simulink model "parallel_prediction_and_cost_function_6phase"  (R2022a)
settings: Solver=FixedStepDiscrete  StartTime=0.0  StopTime=10.0  RelTol=1e-3
undefined symbols (not defined in the file): f_c, L_d, L_q, L_x, L_y, p, psi_pm, R_ph
libraries: hdlsllib x5
(part 2 of 3)

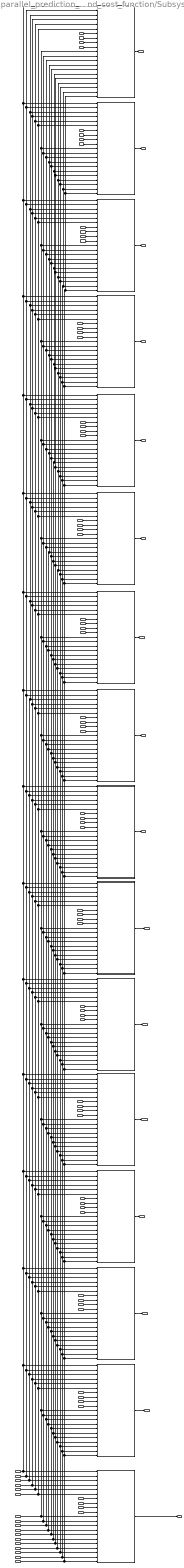
== system parallel_prediction_and_cost_function_6phase/Prediction_and_cost_function/Subsystem ==
  d_phase_voltage_per_switching_state : Inport
  q_phase_voltage_per_switching_state : Inport  Port=2
  x_phase_voltage_per_switching_state : Inport  Port=3
  y_phase_voltage_per_switching_state : Inport  Port=4
  d_phase_voltage_per_switching_state1 : Inport  Port=5
  q_phase_voltage_per_switching_state1 : Inport  Port=6
  x_phase_voltage_per_switching_state1 : Inport  Port=7
  y_phase_voltage_per_switching_state1 : Inport  Port=8
  d_phase_voltage_per_switching_state2 : Inport  Port=9
  q_phase_voltage_per_switching_state2 : Inport  Port=10
  x_phase_voltage_per_switching_state2 : Inport  Port=11
  y_phase_voltage_per_switching_state2 : Inport  Port=12
  d_phase_voltage_per_switching_state3 : Inport  Port=13
  q_phase_voltage_per_switching_state3 : Inport  Port=14
  x_phase_voltage_per_switching_state3 : Inport  Port=15
  y_phase_voltage_per_switching_state3 : Inport  Port=16
  d_phase_voltage_per_switching_state4 : Inport  Port=17
  q_phase_voltage_per_switching_state4 : Inport  Port=18
  x_phase_voltage_per_switching_state4 : Inport  Port=19
  y_phase_voltage_per_switching_state4 : Inport  Port=20
  d_phase_voltage_per_switching_state5 : Inport  Port=21
  q_phase_voltage_per_switching_state5 : Inport  Port=22
  x_phase_voltage_per_switching_state5 : Inport  Port=23
  y_phase_voltage_per_switching_state5 : Inport  Port=24
  d_phase_voltage_per_switching_state6 : Inport  Port=25
  q_phase_voltage_per_switching_state6 : Inport  Port=26
  x_phase_voltage_per_switching_state6 : Inport  Port=27
  y_phase_voltage_per_switching_state6 : Inport  Port=28
  d_phase_voltage_per_switching_state7 : Inport  Port=29
  q_phase_voltage_per_switching_state7 : Inport  Port=30
  x_phase_voltage_per_switching_state7 : Inport  Port=31
  y_phase_voltage_per_switching_state7 : Inport  Port=32
  d_phase_voltage_per_switching_state8 : Inport  Port=33
  q_phase_voltage_per_switching_state8 : Inport  Port=34
  x_phase_voltage_per_switching_state8 : Inport  Port=35
  y_phase_voltage_per_switching_state8 : Inport  Port=36
  d_phase_voltage_per_switching_state9 : Inport  Port=37
  q_phase_voltage_per_switching_state9 : Inport  Port=38
  x_phase_voltage_per_switching_state9 : Inport  Port=39
  y_phase_voltage_per_switching_state9 : Inport  Port=40
  d_phase_voltage_per_switching_state10 : Inport  Port=41
  q_phase_voltage_per_switching_state10 : Inport  Port=42
  x_phase_voltage_per_switching_state10 : Inport  Port=43
  y_phase_voltage_per_switching_state10 : Inport  Port=44
  d_phase_voltage_per_switching_state11 : Inport  Port=45
  q_phase_voltage_per_switching_state11 : Inport  Port=46
  x_phase_voltage_per_switching_state11 : Inport  Port=47
  y_phase_voltage_per_switching_state11 : Inport  Port=48
  d_phase_voltage_per_switching_state12 : Inport  Port=49
  q_phase_voltage_per_switching_state12 : Inport  Port=50
  x_phase_voltage_per_switching_state12 : Inport  Port=51
  y_phase_voltage_per_switching_state12 : Inport  Port=52
  d_phase_voltage_per_switching_state13 : Inport  Port=53
  q_phase_voltage_per_switching_state13 : Inport  Port=54
  x_phase_voltage_per_switching_state13 : Inport  Port=55
  y_phase_voltage_per_switching_state13 : Inport  Port=56
  d_phase_voltage_per_switching_state14 : Inport  Port=57
  q_phase_voltage_per_switching_state14 : Inport  Port=58
  x_phase_voltage_per_switching_state14 : Inport  Port=59
  y_phase_voltage_per_switching_state14 : Inport  Port=60
  SampleTime_div_Ld15 : Inport  Port=61
  SampleTime_div_Lq15 : Inport  Port=62
  SampleTime_div_Lx15 : Inport  Port=63
  SampleTime_div_Ly15 : Inport  Port=64
  id_k_16 : Inport  Port=65
  iq_k_16 : Inport  Port=66
  ix_k_16 : Inport  Port=67
  iy_k_16 : Inport  Port=68
  Rs15 : Inport  Port=69
  omega_el15 : Inport  Port=70
  Lq15 : Inport  Port=71
  Ld15 : Inport  Port=72
  psiPM15 : Inport  Port=73
  d_phase_voltage_per_switching_state15 : Inport  Port=74
  q_phase_voltage_per_switching_state15 : Inport  Port=75
  x_phase_voltage_per_switching_state15 : Inport  Port=76
  y_phase_voltage_per_switching_state15 : Inport  Port=77
  id_ref15 : Inport  Port=78
  iq_ref15 : Inport  Port=79
  ix_ref15 : Inport  Port=80
  iy_ref15 : Inport  Port=81
  Subsystem : Subsystem
  Subsystem1 : Subsystem
  Subsystem10 : Subsystem
  Subsystem11 : Subsystem
  Subsystem12 : Subsystem
  Subsystem13 : Subsystem
  Subsystem14 : Subsystem
  Subsystem15 : Subsystem
  Subsystem2 : Subsystem
  Subsystem3 : Subsystem
  Subsystem4 : Subsystem
  Subsystem5 : Subsystem
  Subsystem6 : Subsystem
  Subsystem7 : Subsystem
  Subsystem8 : Subsystem
  Subsystem9 : Subsystem
  J : Outport
  J1 : Outport  Port=2
  J2 : Outport  Port=3
  J3 : Outport  Port=4
  J4 : Outport  Port=5
  J5 : Outport  Port=6
  J6 : Outport  Port=7
  J7 : Outport  Port=8
  J8 : Outport  Port=9
  J9 : Outport  Port=10
  J10 : Outport  Port=11
  J11 : Outport  Port=12
  J12 : Outport  Port=13
  J13 : Outport  Port=14
  J14 : Outport  Port=15
  J15 : Outport  Port=16
  wires:
  d_phase_voltage_per_switching_state13/1 -> Subsystem2/7(d_phase_voltage_per_switching_state)
  q_phase_voltage_per_switching_state1/1 -> Subsystem14/8(q_phase_voltage_per_switching_state)
  x_phase_voltage_per_switching_state12/1 -> Subsystem3/9(x_phase_voltage_per_switching_state)
  y_phase_voltage_per_switching_state/1 -> Subsystem15/10(y_phase_voltage_per_switching_state)
  y_phase_voltage_per_switching_state2/1 -> Subsystem13/10(y_phase_voltage_per_switching_state)
  d_phase_voltage_per_switching_state1/1 -> Subsystem14/7(d_phase_voltage_per_switching_state)
  x_phase_voltage_per_switching_state1/1 -> Subsystem14/9(x_phase_voltage_per_switching_state)
  y_phase_voltage_per_switching_state7/1 -> Subsystem8/10(y_phase_voltage_per_switching_state)
  d_phase_voltage_per_switching_state3/1 -> Subsystem12/7(d_phase_voltage_per_switching_state)
  d_phase_voltage_per_switching_state6/1 -> Subsystem9/7(d_phase_voltage_per_switching_state)
  x_phase_voltage_per_switching_state9/1 -> Subsystem6/9(x_phase_voltage_per_switching_state)
  d_phase_voltage_per_switching_state/1 -> Subsystem15/7(d_phase_voltage_per_switching_state)
  x_phase_voltage_per_switching_state3/1 -> Subsystem12/9(x_phase_voltage_per_switching_state)
  d_phase_voltage_per_switching_state2/1 -> Subsystem13/7(d_phase_voltage_per_switching_state)
  x_phase_voltage_per_switching_state8/1 -> Subsystem7/9(x_phase_voltage_per_switching_state)
  y_phase_voltage_per_switching_state9/1 -> Subsystem6/10(y_phase_voltage_per_switching_state)
  x_phase_voltage_per_switching_state4/1 -> Subsystem11/9(x_phase_voltage_per_switching_state)
  y_phase_voltage_per_switching_state1/1 -> Subsystem14/10(y_phase_voltage_per_switching_state)
  q_phase_voltage_per_switching_state2/1 -> Subsystem13/8(q_phase_voltage_per_switching_state)
  x_phase_voltage_per_switching_state2/1 -> Subsystem13/9(x_phase_voltage_per_switching_state)
  y_phase_voltage_per_switching_state11/1 -> Subsystem4/10(y_phase_voltage_per_switching_state)
  y_phase_voltage_per_switching_state4/1 -> Subsystem11/10(y_phase_voltage_per_switching_state)
  x_phase_voltage_per_switching_state/1 -> Subsystem15/9(x_phase_voltage_per_switching_state)
  d_phase_voltage_per_switching_state14/1 -> Subsystem1/7(d_phase_voltage_per_switching_state)
  q_phase_voltage_per_switching_state9/1 -> Subsystem6/8(q_phase_voltage_per_switching_state)
  q_phase_voltage_per_switching_state5/1 -> Subsystem10/8(q_phase_voltage_per_switching_state)
  d_phase_voltage_per_switching_state10/1 -> Subsystem5/7(d_phase_voltage_per_switching_state)
  x_phase_voltage_per_switching_state14/1 -> Subsystem1/9(x_phase_voltage_per_switching_state)
  y_phase_voltage_per_switching_state14/1 -> Subsystem1/10(y_phase_voltage_per_switching_state)
  q_phase_voltage_per_switching_state14/1 -> Subsystem1/8(q_phase_voltage_per_switching_state)
  q_phase_voltage_per_switching_state11/1 -> Subsystem4/8(q_phase_voltage_per_switching_state)
  x_phase_voltage_per_switching_state11/1 -> Subsystem4/9(x_phase_voltage_per_switching_state)
  d_phase_voltage_per_switching_state11/1 -> Subsystem4/7(d_phase_voltage_per_switching_state)
  y_phase_voltage_per_switching_state12/1 -> Subsystem3/10(y_phase_voltage_per_switching_state)
  x_phase_voltage_per_switching_state13/1 -> Subsystem2/9(x_phase_voltage_per_switching_state)
  d_phase_voltage_per_switching_state9/1 -> Subsystem6/7(d_phase_voltage_per_switching_state)
  d_phase_voltage_per_switching_state7/1 -> Subsystem8/7(d_phase_voltage_per_switching_state)
  d_phase_voltage_per_switching_state4/1 -> Subsystem11/7(d_phase_voltage_per_switching_state)
  q_phase_voltage_per_switching_state4/1 -> Subsystem11/8(q_phase_voltage_per_switching_state)
  q_phase_voltage_per_switching_state12/1 -> Subsystem3/8(q_phase_voltage_per_switching_state)
  d_phase_voltage_per_switching_state8/1 -> Subsystem7/7(d_phase_voltage_per_switching_state)
  x_phase_voltage_per_switching_state5/1 -> Subsystem10/9(x_phase_voltage_per_switching_state)
  d_phase_voltage_per_switching_state12/1 -> Subsystem3/7(d_phase_voltage_per_switching_state)
  x_phase_voltage_per_switching_state7/1 -> Subsystem8/9(x_phase_voltage_per_switching_state)
  q_phase_voltage_per_switching_state/1 -> Subsystem15/8(q_phase_voltage_per_switching_state)
  d_phase_voltage_per_switching_state5/1 -> Subsystem10/7(d_phase_voltage_per_switching_state)
  q_phase_voltage_per_switching_state13/1 -> Subsystem2/8(q_phase_voltage_per_switching_state)
  y_phase_voltage_per_switching_state5/1 -> Subsystem10/10(y_phase_voltage_per_switching_state)
  q_phase_voltage_per_switching_state6/1 -> Subsystem9/8(q_phase_voltage_per_switching_state)
  y_phase_voltage_per_switching_state6/1 -> Subsystem9/10(y_phase_voltage_per_switching_state)
  x_phase_voltage_per_switching_state6/1 -> Subsystem9/9(x_phase_voltage_per_switching_state)
  y_phase_voltage_per_switching_state8/1 -> Subsystem7/10(y_phase_voltage_per_switching_state)
  q_phase_voltage_per_switching_state8/1 -> Subsystem7/8(q_phase_voltage_per_switching_state)
  y_phase_voltage_per_switching_state13/1 -> Subsystem2/10(y_phase_voltage_per_switching_state)
  q_phase_voltage_per_switching_state7/1 -> Subsystem8/8(q_phase_voltage_per_switching_state)
  x_phase_voltage_per_switching_state10/1 -> Subsystem5/9(x_phase_voltage_per_switching_state)
  q_phase_voltage_per_switching_state10/1 -> Subsystem5/8(q_phase_voltage_per_switching_state)
  y_phase_voltage_per_switching_state10/1 -> Subsystem5/10(y_phase_voltage_per_switching_state)
  y_phase_voltage_per_switching_state3/1 -> Subsystem12/10(y_phase_voltage_per_switching_state)
  q_phase_voltage_per_switching_state3/1 -> Subsystem12/8(q_phase_voltage_per_switching_state)
  id_ref15/1 -> Subsystem15/1(id_ref), Subsystem14/1(id_ref), Subsystem13/1(id_ref), Subsystem12/1(id_ref), Subsystem11/1(id_ref), Subsystem10/1(id_ref), Subsystem9/1(id_ref), Subsystem8/1(id_ref), Subsystem7/1(id_ref), Subsystem6/1(id_ref), Subsystem5/1(id_ref), Subsystem4/1(id_ref), Subsystem3/1(id_ref), Subsystem2/1(id_ref), Subsystem1/1(id_ref), Subsystem/1(id_ref)  "id_ref"
  iq_ref15/1 -> Subsystem/2(iq_ref), Subsystem15/2(iq_ref), Subsystem14/2(iq_ref), Subsystem13/2(iq_ref), Subsystem12/2(iq_ref), Subsystem11/2(iq_ref), Subsystem10/2(iq_ref), Subsystem9/2(iq_ref), Subsystem8/2(iq_ref), Subsystem7/2(iq_ref), Subsystem6/2(iq_ref), Subsystem5/2(iq_ref), Subsystem4/2(iq_ref), Subsystem3/2(iq_ref), Subsystem2/2(iq_ref), Subsystem1/2(iq_ref)  "iq_ref"
  SampleTime_div_Ld15/1 -> Subsystem/3(SampleTime_div_Ld), Subsystem4/3(SampleTime_div_Ld), Subsystem7/3(SampleTime_div_Ld), Subsystem15/3(SampleTime_div_Ld), Subsystem14/3(SampleTime_div_Ld), Subsystem13/3(SampleTime_div_Ld), Subsystem12/3(SampleTime_div_Ld), Subsystem11/3(SampleTime_div_Ld), Subsystem10/3(SampleTime_div_Ld), Subsystem9/3(SampleTime_div_Ld), Subsystem8/3(SampleTime_div_Ld), Subsystem6/3(SampleTime_div_Ld), Subsystem5/3(SampleTime_div_Ld), Subsystem3/3(SampleTime_div_Ld), Subsystem2/3(SampleTime_div_Ld), Subsystem1/3(SampleTime_div_Ld)  "SampleTime_div_Ld"
  SampleTime_div_Lq15/1 -> Subsystem/4(SampleTime_div_Lq), Subsystem4/4(SampleTime_div_Lq), Subsystem15/4(SampleTime_div_Lq), Subsystem14/4(SampleTime_div_Lq), Subsystem13/4(SampleTime_div_Lq), Subsystem12/4(SampleTime_div_Lq), Subsystem11/4(SampleTime_div_Lq), Subsystem10/4(SampleTime_div_Lq), Subsystem9/4(SampleTime_div_Lq), Subsystem8/4(SampleTime_div_Lq), Subsystem7/4(SampleTime_div_Lq), Subsystem6/4(SampleTime_div_Lq), Subsystem5/4(SampleTime_div_Lq), Subsystem3/4(SampleTime_div_Lq), Subsystem2/4(SampleTime_div_Lq), Subsystem1/4(SampleTime_div_Lq)  "SampleTime_div_Lq"
  SampleTime_div_Lx15/1 -> Subsystem/5(SampleTime_div_Lx), Subsystem15/5(SampleTime_div_Lx), Subsystem14/5(SampleTime_div_Lx), Subsystem13/5(SampleTime_div_Lx), Subsystem12/5(SampleTime_div_Lx), Subsystem11/5(SampleTime_div_Lx), Subsystem10/5(SampleTime_div_Lx), Subsystem9/5(SampleTime_div_Lx), Subsystem8/5(SampleTime_div_Lx), Subsystem7/5(SampleTime_div_Lx), Subsystem6/5(SampleTime_div_Lx), Subsystem5/5(SampleTime_div_Lx), Subsystem4/5(SampleTime_div_Lx), Subsystem3/5(SampleTime_div_Lx), Subsystem2/5(SampleTime_div_Lx), Subsystem1/5(SampleTime_div_Lx)  "SampleTime_div_Lx"
  SampleTime_div_Ly15/1 -> Subsystem/6(SampleTime_div_Ly), Subsystem15/6(SampleTime_div_Ly), Subsystem14/6(SampleTime_div_Ly), Subsystem13/6(SampleTime_div_Ly), Subsystem12/6(SampleTime_div_Ly), Subsystem11/6(SampleTime_div_Ly), Subsystem10/6(SampleTime_div_Ly), Subsystem9/6(SampleTime_div_Ly), Subsystem8/6(SampleTime_div_Ly), Subsystem7/6(SampleTime_div_Ly), Subsystem6/6(SampleTime_div_Ly), Subsystem5/6(SampleTime_div_Ly), Subsystem4/6(SampleTime_div_Ly), Subsystem3/6(SampleTime_div_Ly), Subsystem2/6(SampleTime_div_Ly), Subsystem1/6(SampleTime_div_Ly)  "SampleTime_div_Ly"
  d_phase_voltage_per_switching_state15/1 -> Subsystem/7(d_phase_voltage_per_switching_state)
  q_phase_voltage_per_switching_state15/1 -> Subsystem/8(q_phase_voltage_per_switching_state)
  x_phase_voltage_per_switching_state15/1 -> Subsystem/9(x_phase_voltage_per_switching_state)
  y_phase_voltage_per_switching_state15/1 -> Subsystem/10(y_phase_voltage_per_switching_state)
  ix_ref15/1 -> Subsystem/11(ix_ref), Subsystem15/11(ix_ref), Subsystem14/11(ix_ref), Subsystem13/11(ix_ref), Subsystem12/11(ix_ref), Subsystem11/11(ix_ref), Subsystem10/11(ix_ref), Subsystem9/11(ix_ref), Subsystem8/11(ix_ref), Subsystem7/11(ix_ref), Subsystem6/11(ix_ref), Subsystem5/11(ix_ref), Subsystem4/11(ix_ref), Subsystem3/11(ix_ref), Subsystem2/11(ix_ref), Subsystem1/11(ix_ref)  "ix_ref"
  id_k_16/1 -> Subsystem/12(id_k), Subsystem15/12(id_k), Subsystem14/12(id_k), Subsystem13/12(id_k), Subsystem12/12(id_k), Subsystem11/12(id_k), Subsystem10/12(id_k), Subsystem9/12(id_k), Subsystem8/12(id_k), Subsystem7/12(id_k), Subsystem6/12(id_k), Subsystem5/12(id_k), Subsystem4/12(id_k), Subsystem3/12(id_k), Subsystem2/12(id_k), Subsystem1/12(id_k)  "id_k"
  iq_k_16/1 -> Subsystem/13(iq_k), Subsystem15/13(iq_k), Subsystem14/13(iq_k), Subsystem13/13(iq_k), Subsystem12/13(iq_k), Subsystem11/13(iq_k), Subsystem10/13(iq_k), Subsystem9/13(iq_k), Subsystem8/13(iq_k), Subsystem7/13(iq_k), Subsystem6/13(iq_k), Subsystem5/13(iq_k), Subsystem4/13(iq_k), Subsystem3/13(iq_k), Subsystem2/13(iq_k), Subsystem1/13(iq_k)  "iq_k"
  ix_k_16/1 -> Subsystem/14(ix_k), Subsystem15/14(ix_k), Subsystem14/14(ix_k), Subsystem13/14(ix_k), Subsystem12/14(ix_k), Subsystem11/14(ix_k), Subsystem10/14(ix_k), Subsystem9/14(ix_k), Subsystem8/14(ix_k), Subsystem7/14(ix_k), Subsystem6/14(ix_k), Subsystem5/14(ix_k), Subsystem4/14(ix_k), Subsystem3/14(ix_k), Subsystem2/14(ix_k), Subsystem1/14(ix_k)  "ix_k"
  iy_k_16/1 -> Subsystem/15(iy_k), Subsystem15/15(iy_k), Subsystem14/15(iy_k), Subsystem13/15(iy_k), Subsystem12/15(iy_k), Subsystem11/15(iy_k), Subsystem10/15(iy_k), Subsystem9/15(iy_k), Subsystem8/15(iy_k), Subsystem7/15(iy_k), Subsystem6/15(iy_k), Subsystem5/15(iy_k), Subsystem4/15(iy_k), Subsystem3/15(iy_k), Subsystem2/15(iy_k), Subsystem1/15(iy_k)  "iy_k"
  psiPM15/1 -> Subsystem/16(psiPM), Subsystem10/16(psiPM), Subsystem15/16(psiPM), Subsystem14/16(psiPM), Subsystem13/16(psiPM), Subsystem12/16(psiPM), Subsystem11/16(psiPM), Subsystem9/16(psiPM), Subsystem8/16(psiPM), Subsystem7/16(psiPM), Subsystem6/16(psiPM), Subsystem5/16(psiPM), Subsystem4/16(psiPM), Subsystem3/16(psiPM), Subsystem2/16(psiPM), Subsystem1/16(psiPM)  "psiPM"
  Lq15/1 -> Subsystem/17(Lq), Subsystem15/17(Lq), Subsystem14/17(Lq), Subsystem13/17(Lq), Subsystem12/17(Lq), Subsystem11/17(Lq), Subsystem10/17(Lq), Subsystem9/17(Lq), Subsystem8/17(Lq), Subsystem7/17(Lq), Subsystem6/17(Lq), Subsystem5/17(Lq), Subsystem4/17(Lq), Subsystem3/17(Lq), Subsystem2/17(Lq), Subsystem1/17(Lq)  "Lq"
  iy_ref15/1 -> Subsystem/18(iy_ref), Subsystem1/18(iy_ref), Subsystem6/18(iy_ref), Subsystem15/18(iy_ref), Subsystem14/18(iy_ref), Subsystem13/18(iy_ref), Subsystem12/18(iy_ref), Subsystem11/18(iy_ref), Subsystem10/18(iy_ref), Subsystem9/18(iy_ref), Subsystem8/18(iy_ref), Subsystem7/18(iy_ref), Subsystem5/18(iy_ref), Subsystem4/18(iy_ref), Subsystem3/18(iy_ref), Subsystem2/18(iy_ref)  "iy_ref"
  Ld15/1 -> Subsystem/19(Ld), Subsystem1/19(Ld), Subsystem15/19(Ld), Subsystem14/19(Ld), Subsystem13/19(Ld), Subsystem12/19(Ld), Subsystem11/19(Ld), Subsystem10/19(Ld), Subsystem9/19(Ld), Subsystem8/19(Ld), Subsystem7/19(Ld), Subsystem6/19(Ld), Subsystem5/19(Ld), Subsystem4/19(Ld), Subsystem3/19(Ld), Subsystem2/19(Ld)  "Ld"
  Rs15/1 -> Subsystem/20(Rs), Subsystem7/20(Rs), Subsystem15/20(Rs), Subsystem14/20(Rs), Subsystem13/20(Rs), Subsystem12/20(Rs), Subsystem11/20(Rs), Subsystem10/20(Rs), Subsystem9/20(Rs), Subsystem8/20(Rs), Subsystem6/20(Rs), Subsystem5/20(Rs), Subsystem4/20(Rs), Subsystem3/20(Rs), Subsystem2/20(Rs), Subsystem1/20(Rs)  "Rs"
  omega_el15/1 -> Subsystem/21(omega_el), Subsystem15/21(omega_el), Subsystem14/21(omega_el), Subsystem13/21(omega_el), Subsystem12/21(omega_el), Subsystem11/21(omega_el), Subsystem10/21(omega_el), Subsystem9/21(omega_el), Subsystem8/21(omega_el), Subsystem7/21(omega_el), Subsystem6/21(omega_el), Subsystem5/21(omega_el), Subsystem4/21(omega_el), Subsystem3/21(omega_el), Subsystem2/21(omega_el), Subsystem1/21(omega_el)  "omega_el"
  Subsystem/1(J15) -> J15/1
  Subsystem1/1(J) -> J14/1
  Subsystem2/1(J) -> J13/1
  Subsystem3/1(J) -> J12/1
  Subsystem4/1(J) -> J11/1
  Subsystem5/1(J) -> J10/1
  Subsystem6/1(J) -> J9/1
  Subsystem7/1(J) -> J8/1
  Subsystem8/1(J) -> J7/1
  Subsystem9/1(J) -> J6/1
  Subsystem10/1(J) -> J5/1
  Subsystem11/1(J) -> J4/1
  Subsystem12/1(J) -> J3/1
  Subsystem13/1(J) -> J2/1
  Subsystem14/1(J) -> J1/1
  Subsystem15/1(J) -> J/1

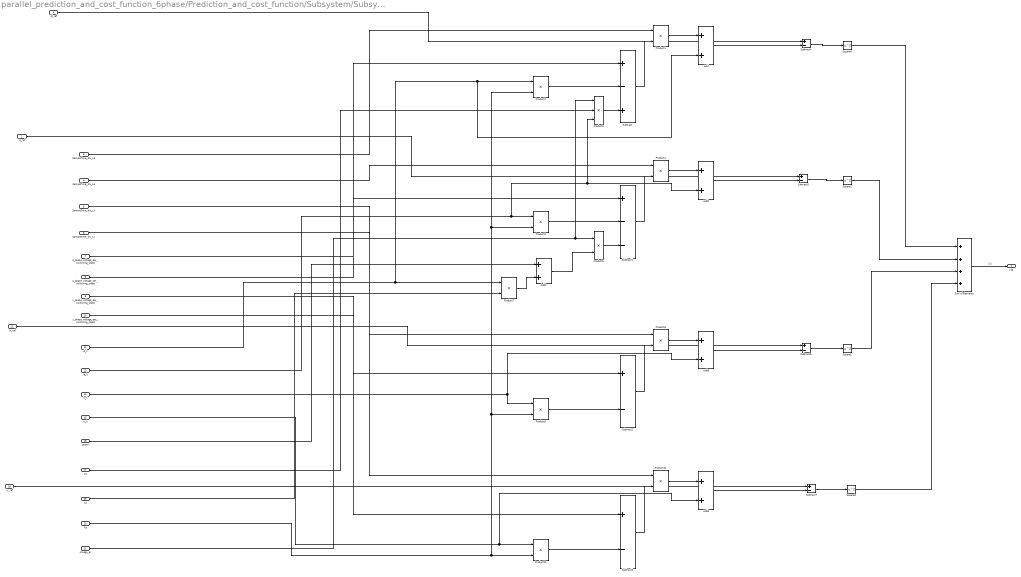
== system parallel_prediction_and_cost_function_6phase/Prediction_and_cost_function/Subsystem/Subsystem ==
  id_ref : Inport
  iq_ref : Inport  Port=2
  SampleTime_div_Ld : Inport  Port=3
  SampleTime_div_Lq : Inport  Port=4
  SampleTime_div_Lx : Inport  Port=5
  SampleTime_div_Ly : Inport  Port=6
  d_phase_voltage_per_switching_state : Inport  Port=7
  q_phase_voltage_per_switching_state : Inport  Port=8
  x_phase_voltage_per_switching_state : Inport  Port=9
  y_phase_voltage_per_switching_state : Inport  Port=10
  ix_ref : Inport  Port=11
  id_k : Inport  Port=12
  iq_k : Inport  Port=13
  ix_k : Inport  Port=14
  iy_k : Inport  Port=15
  psiPM : Inport  Port=16
  Lq : Inport  Port=17
  iy_ref : Inport  Port=18
  Ld : Inport  Port=19
  Rs : Inport  Port=20
  omega_el : Inport  Port=21
  Add{,1,3..4} (4 alike) : Sum  OutDataTypeStr=single
  Add2 : Sum
  Product{1..2,4..11} (10 alike) : Product  OutDataTypeStr=single
  Product3 : Product  Inputs=3  OutDataTypeStr=single
  Square{1..4} (4 alike) : Math  Operator=square  SignedPower=on  RndMeth=Zero
  Subtract : Sum  Inputs=+-+  OutDataTypeStr=single
  Subtract1 : Sum  Inputs=+--  OutDataTypeStr=single
  Subtract2 : Sum  Inputs=+-  OutDataTypeStr=single
  Subtract3 : Sum  Inputs=+-  OutDataTypeStr=single
  Subtract{4..7} (4 alike) : Sum  Inputs=+-
  Sum of Elements : Sum  Inputs=++++
  J15 : Outport
  wires:
  Add1/1 -> Subtract5/2
  q_phase_voltage_per_switching_state/1 -> Subtract1/1
  ix_ref/1 -> Subtract6/1
  omega_el/1 -> Product3/1, Product6/1
  Product5/1 -> Subtract1/2
  iq_k/1 -> Product3/3, Add1/2, Product5/1
  iy_k/1 -> Add4/2, Product11/1
  Add2/1 -> Product6/2
  Lq/1 -> Product3/2
  Add4/1 -> Subtract7/2
  Subtract2/1 -> Product8/2
  SampleTime_div_Ly/1 -> Product10/1
  Rs/1 -> Product9/2, Product2/2, Product5/2, Product11/2
  Product9/1 -> Subtract2/2
  Product8/1 -> Add3/1
  Product7/1 -> Add2/2
  id_k/1 -> Add/2, Product2/1, Product7/1
  x_phase_voltage_per_switching_state/1 -> Subtract2/1
  Add3/1 -> Subtract6/2
  Add/1 -> Subtract4/2
  Product11/1 -> Subtract3/2
  Product6/1 -> Subtract1/3
  Subtract1/1 -> Product4/2
  Product1/1 -> Add/1
  Product10/1 -> Add4/1
  Product4/1 -> Add1/1
  SampleTime_div_Ld/1 -> Product1/1
  y_phase_voltage_per_switching_state/1 -> Subtract3/1
  Product2/1 -> Subtract/2
  Subtract5/1 -> Square1/1
  Product3/1 -> Subtract/3
  SampleTime_div_Lq/1 -> Product4/1
  Subtract/1 -> Product1/2
  Subtract3/1 -> Product10/2
  Sum of Elements/1 -> J15/1  "J15"
  psiPM/1 -> Add2/1
  id_ref/1 -> Subtract4/1
  Subtract6/1 -> Square2/1
  Ld/1 -> Product7/2
  iy_ref/1 -> Subtract7/1
  ix_k/1 -> Add3/2, Product9/1
  Subtract4/1 -> Square4/1
  Subtract7/1 -> Square3/1
  iq_ref/1 -> Subtract5/1
  SampleTime_div_Lx/1 -> Product8/1
  d_phase_voltage_per_switching_state/1 -> Subtract/1
  Square3/1 -> Sum of Elements/4
  Square2/1 -> Sum of Elements/3
  Square1/1 -> Sum of Elements/2
  Square4/1 -> Sum of Elements/1

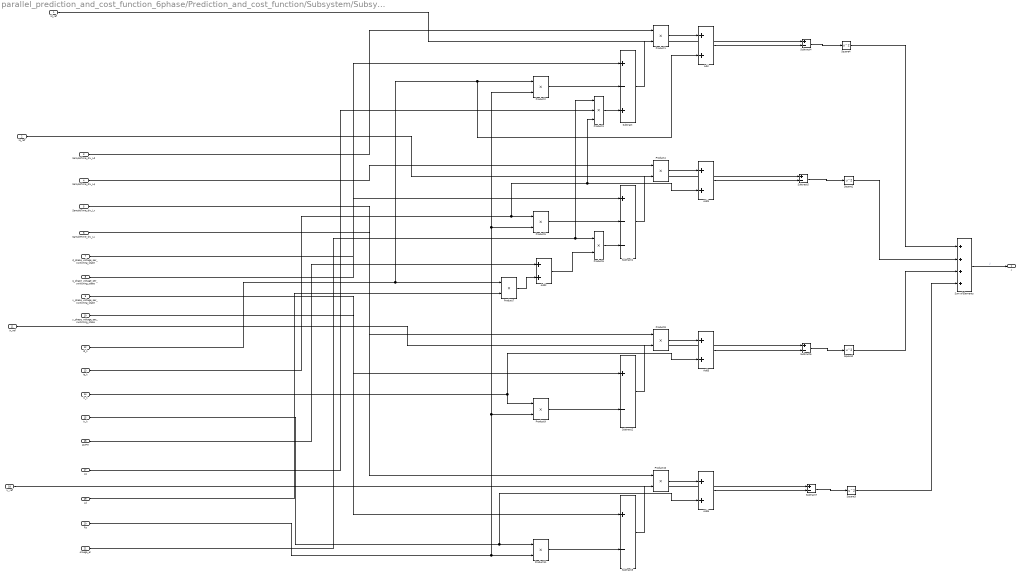
== system parallel_prediction_and_cost_function_6phase/Prediction_and_cost_function/Subsystem/Subsystem1 ==
  id_ref : Inport
  iq_ref : Inport  Port=2
  SampleTime_div_Ld : Inport  Port=3
  SampleTime_div_Lq : Inport  Port=4
  SampleTime_div_Lx : Inport  Port=5
  SampleTime_div_Ly : Inport  Port=6
  d_phase_voltage_per_switching_state : Inport  Port=7
  q_phase_voltage_per_switching_state : Inport  Port=8
  x_phase_voltage_per_switching_state : Inport  Port=9
  y_phase_voltage_per_switching_state : Inport  Port=10
  ix_ref : Inport  Port=11
  id_k : Inport  Port=12
  iq_k : Inport  Port=13
  ix_k : Inport  Port=14
  iy_k : Inport  Port=15
  psiPM : Inport  Port=16
  Lq : Inport  Port=17
  iy_ref : Inport  Port=18
  Ld : Inport  Port=19
  Rs : Inport  Port=20
  omega_el : Inport  Port=21
  Add{,1,3..4} (4 alike) : Sum  OutDataTypeStr=single
  Add2 : Sum
  Product{1..2,4..11} (10 alike) : Product  OutDataTypeStr=single
  Product3 : Product  Inputs=3  OutDataTypeStr=single
  Square{1..4} (4 alike) : Math  Operator=square  SignedPower=on  RndMeth=Zero
  Subtract : Sum  Inputs=+-+  OutDataTypeStr=single
  Subtract1 : Sum  Inputs=+--  OutDataTypeStr=single
  Subtract2 : Sum  Inputs=+-  OutDataTypeStr=single
  Subtract3 : Sum  Inputs=+-  OutDataTypeStr=single
  Subtract{4..7} (4 alike) : Sum  Inputs=+-
  Sum of Elements : Sum  Inputs=++++
  J : Outport
  wires:
  Add1/1 -> Subtract5/2
  q_phase_voltage_per_switching_state/1 -> Subtract1/1
  ix_ref/1 -> Subtract6/1
  omega_el/1 -> Product3/1, Product6/1
  Product5/1 -> Subtract1/2
  iq_k/1 -> Product3/3, Add1/2, Product5/1
  iy_k/1 -> Add4/2, Product11/1
  Add2/1 -> Product6/2
  Lq/1 -> Product3/2
  Add4/1 -> Subtract7/2
  Subtract2/1 -> Product8/2
  SampleTime_div_Ly/1 -> Product10/1
  Rs/1 -> Product9/2, Product2/2, Product5/2, Product11/2
  Product9/1 -> Subtract2/2
  Product8/1 -> Add3/1
  Product7/1 -> Add2/2
  id_k/1 -> Add/2, Product2/1, Product7/1
  x_phase_voltage_per_switching_state/1 -> Subtract2/1
  Add3/1 -> Subtract6/2
  Add/1 -> Subtract4/2
  Product11/1 -> Subtract3/2
  Product6/1 -> Subtract1/3
  Subtract1/1 -> Product4/2
  Product1/1 -> Add/1
  Product10/1 -> Add4/1
  Product4/1 -> Add1/1
  SampleTime_div_Ld/1 -> Product1/1
  y_phase_voltage_per_switching_state/1 -> Subtract3/1
  Product2/1 -> Subtract/2
  Subtract5/1 -> Square1/1
  Product3/1 -> Subtract/3
  SampleTime_div_Lq/1 -> Product4/1
  Subtract/1 -> Product1/2
  Subtract3/1 -> Product10/2
  Sum of Elements/1 -> J/1  "J"
  psiPM/1 -> Add2/1
  id_ref/1 -> Subtract4/1
  Subtract6/1 -> Square2/1
  Ld/1 -> Product7/2
  iy_ref/1 -> Subtract7/1
  ix_k/1 -> Add3/2, Product9/1
  Subtract4/1 -> Square4/1
  Subtract7/1 -> Square3/1
  iq_ref/1 -> Subtract5/1
  SampleTime_div_Lx/1 -> Product8/1
  d_phase_voltage_per_switching_state/1 -> Subtract/1
  Square3/1 -> Sum of Elements/4
  Square2/1 -> Sum of Elements/3
  Square1/1 -> Sum of Elements/2
  Square4/1 -> Sum of Elements/1

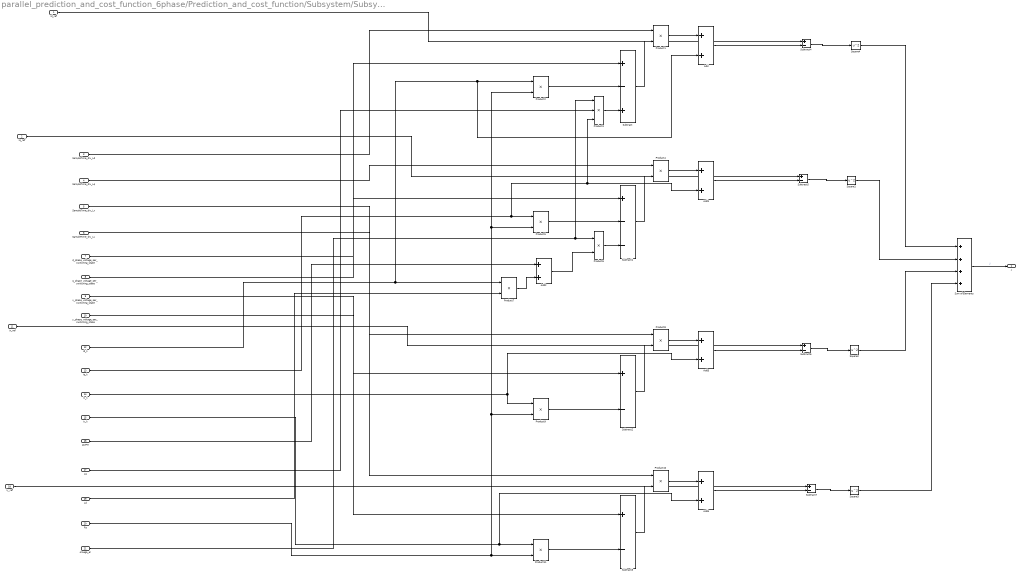
== system parallel_prediction_and_cost_function_6phase/Prediction_and_cost_function/Subsystem/Subsystem10 ==
  id_ref : Inport
  iq_ref : Inport  Port=2
  SampleTime_div_Ld : Inport  Port=3
  SampleTime_div_Lq : Inport  Port=4
  SampleTime_div_Lx : Inport  Port=5
  SampleTime_div_Ly : Inport  Port=6
  d_phase_voltage_per_switching_state : Inport  Port=7
  q_phase_voltage_per_switching_state : Inport  Port=8
  x_phase_voltage_per_switching_state : Inport  Port=9
  y_phase_voltage_per_switching_state : Inport  Port=10
  ix_ref : Inport  Port=11
  id_k : Inport  Port=12
  iq_k : Inport  Port=13
  ix_k : Inport  Port=14
  iy_k : Inport  Port=15
  psiPM : Inport  Port=16
  Lq : Inport  Port=17
  iy_ref : Inport  Port=18
  Ld : Inport  Port=19
  Rs : Inport  Port=20
  omega_el : Inport  Port=21
  Add{,1,3..4} (4 alike) : Sum  OutDataTypeStr=single
  Add2 : Sum
  Product{1..2,4..11} (10 alike) : Product  OutDataTypeStr=single
  Product3 : Product  Inputs=3  OutDataTypeStr=single
  Square{1..4} (4 alike) : Math  Operator=square  SignedPower=on  RndMeth=Zero
  Subtract : Sum  Inputs=+-+  OutDataTypeStr=single
  Subtract1 : Sum  Inputs=+--  OutDataTypeStr=single
  Subtract2 : Sum  Inputs=+-  OutDataTypeStr=single
  Subtract3 : Sum  Inputs=+-  OutDataTypeStr=single
  Subtract{4..7} (4 alike) : Sum  Inputs=+-
  Sum of Elements : Sum  Inputs=++++
  J : Outport
  wires:
  Add1/1 -> Subtract5/2
  q_phase_voltage_per_switching_state/1 -> Subtract1/1
  ix_ref/1 -> Subtract6/1
  omega_el/1 -> Product3/1, Product6/1
  Product5/1 -> Subtract1/2
  iq_k/1 -> Product3/3, Add1/2, Product5/1
  iy_k/1 -> Add4/2, Product11/1
  Add2/1 -> Product6/2
  Lq/1 -> Product3/2
  Add4/1 -> Subtract7/2
  Subtract2/1 -> Product8/2
  SampleTime_div_Ly/1 -> Product10/1
  Rs/1 -> Product9/2, Product2/2, Product5/2, Product11/2
  Product9/1 -> Subtract2/2
  Product8/1 -> Add3/1
  Product7/1 -> Add2/2
  id_k/1 -> Add/2, Product2/1, Product7/1
  x_phase_voltage_per_switching_state/1 -> Subtract2/1
  Add3/1 -> Subtract6/2
  Add/1 -> Subtract4/2
  Product11/1 -> Subtract3/2
  Product6/1 -> Subtract1/3
  Subtract1/1 -> Product4/2
  Product1/1 -> Add/1
  Product10/1 -> Add4/1
  Product4/1 -> Add1/1
  SampleTime_div_Ld/1 -> Product1/1
  y_phase_voltage_per_switching_state/1 -> Subtract3/1
  Product2/1 -> Subtract/2
  Subtract5/1 -> Square1/1
  Product3/1 -> Subtract/3
  SampleTime_div_Lq/1 -> Product4/1
  Subtract/1 -> Product1/2
  Subtract3/1 -> Product10/2
  Sum of Elements/1 -> J/1  "J"
  psiPM/1 -> Add2/1
  id_ref/1 -> Subtract4/1
  Subtract6/1 -> Square2/1
  Ld/1 -> Product7/2
  iy_ref/1 -> Subtract7/1
  ix_k/1 -> Add3/2, Product9/1
  Subtract4/1 -> Square4/1
  Subtract7/1 -> Square3/1
  iq_ref/1 -> Subtract5/1
  SampleTime_div_Lx/1 -> Product8/1
  d_phase_voltage_per_switching_state/1 -> Subtract/1
  Square3/1 -> Sum of Elements/4
  Square2/1 -> Sum of Elements/3
  Square1/1 -> Sum of Elements/2
  Square4/1 -> Sum of Elements/1

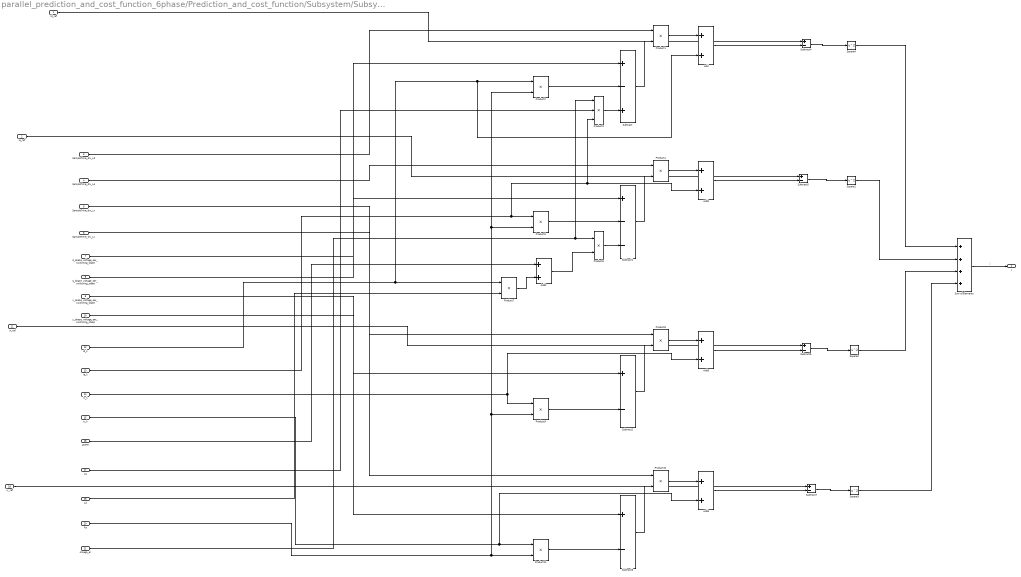
== system parallel_prediction_and_cost_function_6phase/Prediction_and_cost_function/Subsystem/Subsystem11 ==
  id_ref : Inport
  iq_ref : Inport  Port=2
  SampleTime_div_Ld : Inport  Port=3
  SampleTime_div_Lq : Inport  Port=4
  SampleTime_div_Lx : Inport  Port=5
  SampleTime_div_Ly : Inport  Port=6
  d_phase_voltage_per_switching_state : Inport  Port=7
  q_phase_voltage_per_switching_state : Inport  Port=8
  x_phase_voltage_per_switching_state : Inport  Port=9
  y_phase_voltage_per_switching_state : Inport  Port=10
  ix_ref : Inport  Port=11
  id_k : Inport  Port=12
  iq_k : Inport  Port=13
  ix_k : Inport  Port=14
  iy_k : Inport  Port=15
  psiPM : Inport  Port=16
  Lq : Inport  Port=17
  iy_ref : Inport  Port=18
  Ld : Inport  Port=19
  Rs : Inport  Port=20
  omega_el : Inport  Port=21
  Add{,1,3..4} (4 alike) : Sum  OutDataTypeStr=single
  Add2 : Sum
  Product{1..2,4..11} (10 alike) : Product  OutDataTypeStr=single
  Product3 : Product  Inputs=3  OutDataTypeStr=single
  Square{1..4} (4 alike) : Math  Operator=square  SignedPower=on  RndMeth=Zero
  Subtract : Sum  Inputs=+-+  OutDataTypeStr=single
  Subtract1 : Sum  Inputs=+--  OutDataTypeStr=single
  Subtract2 : Sum  Inputs=+-  OutDataTypeStr=single
  Subtract3 : Sum  Inputs=+-  OutDataTypeStr=single
  Subtract{4..7} (4 alike) : Sum  Inputs=+-
  Sum of Elements : Sum  Inputs=++++
  J : Outport
  wires:
  Add1/1 -> Subtract5/2
  q_phase_voltage_per_switching_state/1 -> Subtract1/1
  ix_ref/1 -> Subtract6/1
  omega_el/1 -> Product3/1, Product6/1
  Product5/1 -> Subtract1/2
  iq_k/1 -> Product3/3, Add1/2, Product5/1
  iy_k/1 -> Add4/2, Product11/1
  Add2/1 -> Product6/2
  Lq/1 -> Product3/2
  Add4/1 -> Subtract7/2
  Subtract2/1 -> Product8/2
  SampleTime_div_Ly/1 -> Product10/1
  Rs/1 -> Product9/2, Product2/2, Product5/2, Product11/2
  Product9/1 -> Subtract2/2
  Product8/1 -> Add3/1
  Product7/1 -> Add2/2
  id_k/1 -> Add/2, Product2/1, Product7/1
  x_phase_voltage_per_switching_state/1 -> Subtract2/1
  Add3/1 -> Subtract6/2
  Add/1 -> Subtract4/2
  Product11/1 -> Subtract3/2
  Product6/1 -> Subtract1/3
  Subtract1/1 -> Product4/2
  Product1/1 -> Add/1
  Product10/1 -> Add4/1
  Product4/1 -> Add1/1
  SampleTime_div_Ld/1 -> Product1/1
  y_phase_voltage_per_switching_state/1 -> Subtract3/1
  Product2/1 -> Subtract/2
  Subtract5/1 -> Square1/1
  Product3/1 -> Subtract/3
  SampleTime_div_Lq/1 -> Product4/1
  Subtract/1 -> Product1/2
  Subtract3/1 -> Product10/2
  Sum of Elements/1 -> J/1  "J"
  psiPM/1 -> Add2/1
  id_ref/1 -> Subtract4/1
  Subtract6/1 -> Square2/1
  Ld/1 -> Product7/2
  iy_ref/1 -> Subtract7/1
  ix_k/1 -> Add3/2, Product9/1
  Subtract4/1 -> Square4/1
  Subtract7/1 -> Square3/1
  iq_ref/1 -> Subtract5/1
  SampleTime_div_Lx/1 -> Product8/1
  d_phase_voltage_per_switching_state/1 -> Subtract/1
  Square3/1 -> Sum of Elements/4
  Square2/1 -> Sum of Elements/3
  Square1/1 -> Sum of Elements/2
  Square4/1 -> Sum of Elements/1

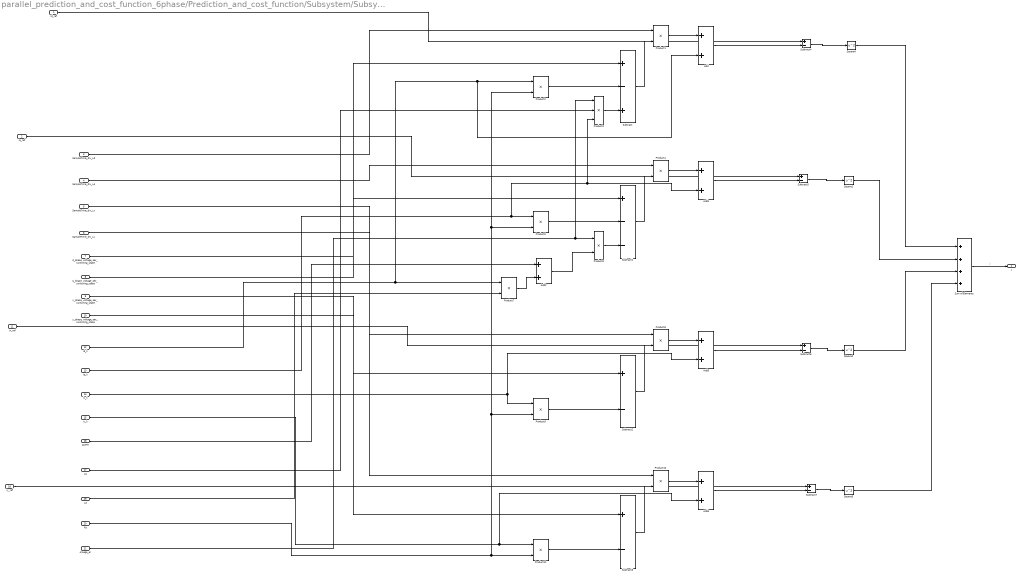
== system parallel_prediction_and_cost_function_6phase/Prediction_and_cost_function/Subsystem/Subsystem12 ==
  id_ref : Inport
  iq_ref : Inport  Port=2
  SampleTime_div_Ld : Inport  Port=3
  SampleTime_div_Lq : Inport  Port=4
  SampleTime_div_Lx : Inport  Port=5
  SampleTime_div_Ly : Inport  Port=6
  d_phase_voltage_per_switching_state : Inport  Port=7
  q_phase_voltage_per_switching_state : Inport  Port=8
  x_phase_voltage_per_switching_state : Inport  Port=9
  y_phase_voltage_per_switching_state : Inport  Port=10
  ix_ref : Inport  Port=11
  id_k : Inport  Port=12
  iq_k : Inport  Port=13
  ix_k : Inport  Port=14
  iy_k : Inport  Port=15
  psiPM : Inport  Port=16
  Lq : Inport  Port=17
  iy_ref : Inport  Port=18
  Ld : Inport  Port=19
  Rs : Inport  Port=20
  omega_el : Inport  Port=21
  Add{,1,3..4} (4 alike) : Sum  OutDataTypeStr=single
  Add2 : Sum
  Product{1..2,4..11} (10 alike) : Product  OutDataTypeStr=single
  Product3 : Product  Inputs=3  OutDataTypeStr=single
  Square{1..4} (4 alike) : Math  Operator=square  SignedPower=on  RndMeth=Zero
  Subtract : Sum  Inputs=+-+  OutDataTypeStr=single
  Subtract1 : Sum  Inputs=+--  OutDataTypeStr=single
  Subtract2 : Sum  Inputs=+-  OutDataTypeStr=single
  Subtract3 : Sum  Inputs=+-  OutDataTypeStr=single
  Subtract{4..7} (4 alike) : Sum  Inputs=+-
  Sum of Elements : Sum  Inputs=++++
  J : Outport
  wires:
  Add1/1 -> Subtract5/2
  q_phase_voltage_per_switching_state/1 -> Subtract1/1
  ix_ref/1 -> Subtract6/1
  omega_el/1 -> Product3/1, Product6/1
  Product5/1 -> Subtract1/2
  iq_k/1 -> Product3/3, Add1/2, Product5/1
  iy_k/1 -> Add4/2, Product11/1
  Add2/1 -> Product6/2
  Lq/1 -> Product3/2
  Add4/1 -> Subtract7/2
  Subtract2/1 -> Product8/2
  SampleTime_div_Ly/1 -> Product10/1
  Rs/1 -> Product9/2, Product2/2, Product5/2, Product11/2
  Product9/1 -> Subtract2/2
  Product8/1 -> Add3/1
  Product7/1 -> Add2/2
  id_k/1 -> Add/2, Product2/1, Product7/1
  x_phase_voltage_per_switching_state/1 -> Subtract2/1
  Add3/1 -> Subtract6/2
  Add/1 -> Subtract4/2
  Product11/1 -> Subtract3/2
  Product6/1 -> Subtract1/3
  Subtract1/1 -> Product4/2
  Product1/1 -> Add/1
  Product10/1 -> Add4/1
  Product4/1 -> Add1/1
  SampleTime_div_Ld/1 -> Product1/1
  y_phase_voltage_per_switching_state/1 -> Subtract3/1
  Product2/1 -> Subtract/2
  Subtract5/1 -> Square1/1
  Product3/1 -> Subtract/3
  SampleTime_div_Lq/1 -> Product4/1
  Subtract/1 -> Product1/2
  Subtract3/1 -> Product10/2
  Sum of Elements/1 -> J/1  "J"
  psiPM/1 -> Add2/1
  id_ref/1 -> Subtract4/1
  Subtract6/1 -> Square2/1
  Ld/1 -> Product7/2
  iy_ref/1 -> Subtract7/1
  ix_k/1 -> Add3/2, Product9/1
  Subtract4/1 -> Square4/1
  Subtract7/1 -> Square3/1
  iq_ref/1 -> Subtract5/1
  SampleTime_div_Lx/1 -> Product8/1
  d_phase_voltage_per_switching_state/1 -> Subtract/1
  Square3/1 -> Sum of Elements/4
  Square2/1 -> Sum of Elements/3
  Square1/1 -> Sum of Elements/2
  Square4/1 -> Sum of Elements/1

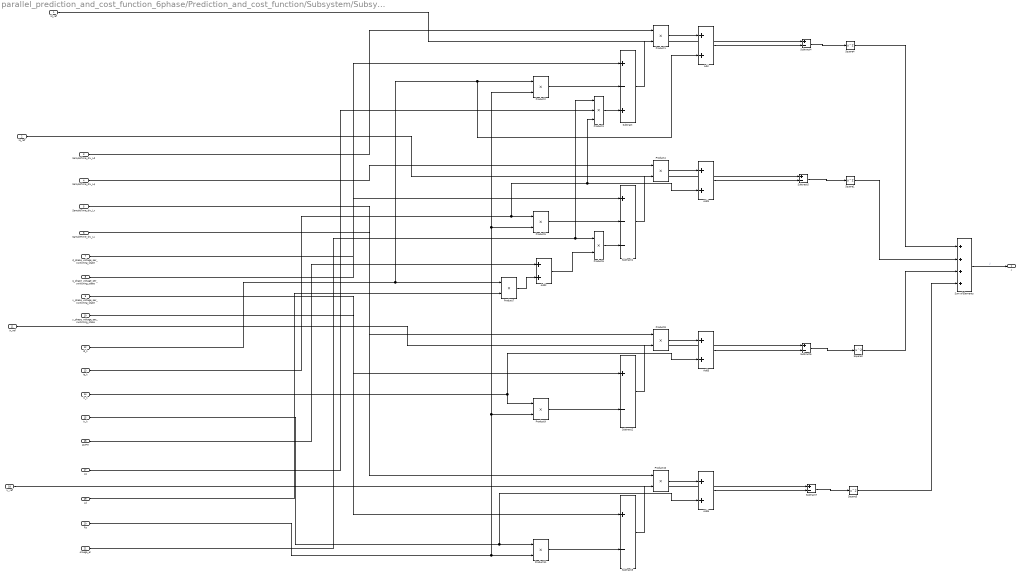
== system parallel_prediction_and_cost_function_6phase/Prediction_and_cost_function/Subsystem/Subsystem13 ==
  id_ref : Inport
  iq_ref : Inport  Port=2
  SampleTime_div_Ld : Inport  Port=3
  SampleTime_div_Lq : Inport  Port=4
  SampleTime_div_Lx : Inport  Port=5
  SampleTime_div_Ly : Inport  Port=6
  d_phase_voltage_per_switching_state : Inport  Port=7
  q_phase_voltage_per_switching_state : Inport  Port=8
  x_phase_voltage_per_switching_state : Inport  Port=9
  y_phase_voltage_per_switching_state : Inport  Port=10
  ix_ref : Inport  Port=11
  id_k : Inport  Port=12
  iq_k : Inport  Port=13
  ix_k : Inport  Port=14
  iy_k : Inport  Port=15
  psiPM : Inport  Port=16
  Lq : Inport  Port=17
  iy_ref : Inport  Port=18
  Ld : Inport  Port=19
  Rs : Inport  Port=20
  omega_el : Inport  Port=21
  Add{,1,3..4} (4 alike) : Sum  OutDataTypeStr=single
  Add2 : Sum
  Product{1..2,4..11} (10 alike) : Product  OutDataTypeStr=single
  Product3 : Product  Inputs=3  OutDataTypeStr=single
  Square{1..4} (4 alike) : Math  Operator=square  SignedPower=on  RndMeth=Zero
  Subtract : Sum  Inputs=+-+  OutDataTypeStr=single
  Subtract1 : Sum  Inputs=+--  OutDataTypeStr=single
  Subtract2 : Sum  Inputs=+-  OutDataTypeStr=single
  Subtract3 : Sum  Inputs=+-  OutDataTypeStr=single
  Subtract{4..7} (4 alike) : Sum  Inputs=+-
  Sum of Elements : Sum  Inputs=++++
  J : Outport
  wires:
  Add1/1 -> Subtract5/2
  q_phase_voltage_per_switching_state/1 -> Subtract1/1
  ix_ref/1 -> Subtract6/1
  omega_el/1 -> Product3/1, Product6/1
  Product5/1 -> Subtract1/2
  iq_k/1 -> Product3/3, Add1/2, Product5/1
  iy_k/1 -> Add4/2, Product11/1
  Add2/1 -> Product6/2
  Lq/1 -> Product3/2
  Add4/1 -> Subtract7/2
  Subtract2/1 -> Product8/2
  SampleTime_div_Ly/1 -> Product10/1
  Rs/1 -> Product9/2, Product2/2, Product5/2, Product11/2
  Product9/1 -> Subtract2/2
  Product8/1 -> Add3/1
  Product7/1 -> Add2/2
  id_k/1 -> Add/2, Product2/1, Product7/1
  x_phase_voltage_per_switching_state/1 -> Subtract2/1
  Add3/1 -> Subtract6/2
  Add/1 -> Subtract4/2
  Product11/1 -> Subtract3/2
  Product6/1 -> Subtract1/3
  Subtract1/1 -> Product4/2
  Product1/1 -> Add/1
  Product10/1 -> Add4/1
  Product4/1 -> Add1/1
  SampleTime_div_Ld/1 -> Product1/1
  y_phase_voltage_per_switching_state/1 -> Subtract3/1
  Product2/1 -> Subtract/2
  Subtract5/1 -> Square1/1
  Product3/1 -> Subtract/3
  SampleTime_div_Lq/1 -> Product4/1
  Subtract/1 -> Product1/2
  Subtract3/1 -> Product10/2
  Sum of Elements/1 -> J/1  "J"
  psiPM/1 -> Add2/1
  id_ref/1 -> Subtract4/1
  Subtract6/1 -> Square2/1
  Ld/1 -> Product7/2
  iy_ref/1 -> Subtract7/1
  ix_k/1 -> Add3/2, Product9/1
  Subtract4/1 -> Square4/1
  Subtract7/1 -> Square3/1
  iq_ref/1 -> Subtract5/1
  SampleTime_div_Lx/1 -> Product8/1
  d_phase_voltage_per_switching_state/1 -> Subtract/1
  Square3/1 -> Sum of Elements/4
  Square2/1 -> Sum of Elements/3
  Square1/1 -> Sum of Elements/2
  Square4/1 -> Sum of Elements/1

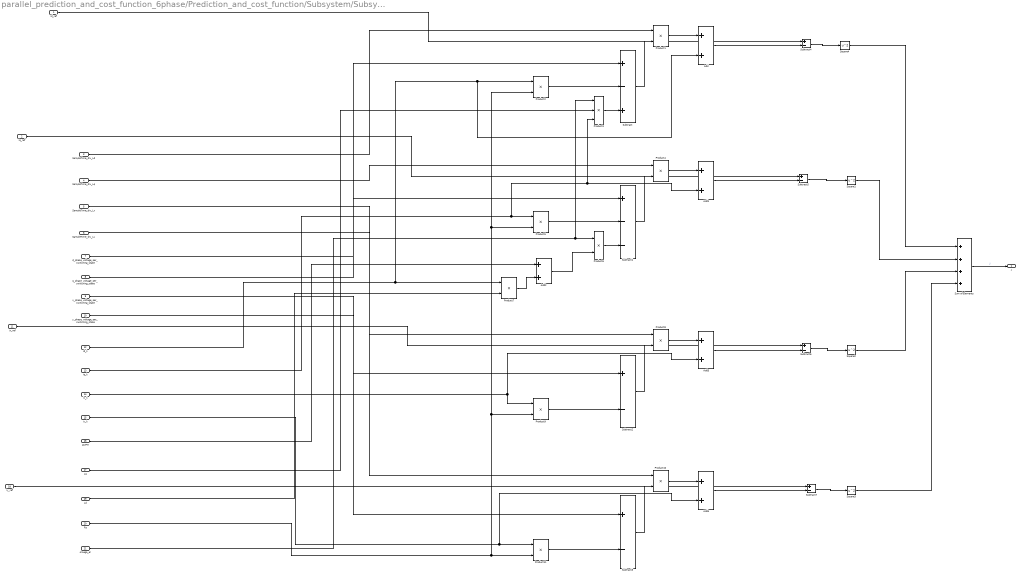
== system parallel_prediction_and_cost_function_6phase/Prediction_and_cost_function/Subsystem/Subsystem14 ==
  id_ref : Inport
  iq_ref : Inport  Port=2
  SampleTime_div_Ld : Inport  Port=3
  SampleTime_div_Lq : Inport  Port=4
  SampleTime_div_Lx : Inport  Port=5
  SampleTime_div_Ly : Inport  Port=6
  d_phase_voltage_per_switching_state : Inport  Port=7
  q_phase_voltage_per_switching_state : Inport  Port=8
  x_phase_voltage_per_switching_state : Inport  Port=9
  y_phase_voltage_per_switching_state : Inport  Port=10
  ix_ref : Inport  Port=11
  id_k : Inport  Port=12
  iq_k : Inport  Port=13
  ix_k : Inport  Port=14
  iy_k : Inport  Port=15
  psiPM : Inport  Port=16
  Lq : Inport  Port=17
  iy_ref : Inport  Port=18
  Ld : Inport  Port=19
  Rs : Inport  Port=20
  omega_el : Inport  Port=21
  Add{,1,3..4} (4 alike) : Sum  OutDataTypeStr=single
  Add2 : Sum
  Product{1..2,4..11} (10 alike) : Product  OutDataTypeStr=single
  Product3 : Product  Inputs=3  OutDataTypeStr=single
  Square{1..4} (4 alike) : Math  Operator=square  SignedPower=on  RndMeth=Zero
  Subtract : Sum  Inputs=+-+  OutDataTypeStr=single
  Subtract1 : Sum  Inputs=+--  OutDataTypeStr=single
  Subtract2 : Sum  Inputs=+-  OutDataTypeStr=single
  Subtract3 : Sum  Inputs=+-  OutDataTypeStr=single
  Subtract{4..7} (4 alike) : Sum  Inputs=+-
  Sum of Elements : Sum  Inputs=++++
  J : Outport
  wires:
  Add1/1 -> Subtract5/2
  q_phase_voltage_per_switching_state/1 -> Subtract1/1
  ix_ref/1 -> Subtract6/1
  omega_el/1 -> Product3/1, Product6/1
  Product5/1 -> Subtract1/2
  iq_k/1 -> Product3/3, Add1/2, Product5/1
  iy_k/1 -> Add4/2, Product11/1
  Add2/1 -> Product6/2
  Lq/1 -> Product3/2
  Add4/1 -> Subtract7/2
  Subtract2/1 -> Product8/2
  SampleTime_div_Ly/1 -> Product10/1
  Rs/1 -> Product9/2, Product2/2, Product5/2, Product11/2
  Product9/1 -> Subtract2/2
  Product8/1 -> Add3/1
  Product7/1 -> Add2/2
  id_k/1 -> Add/2, Product2/1, Product7/1
  x_phase_voltage_per_switching_state/1 -> Subtract2/1
  Add3/1 -> Subtract6/2
  Add/1 -> Subtract4/2
  Product11/1 -> Subtract3/2
  Product6/1 -> Subtract1/3
  Subtract1/1 -> Product4/2
  Product1/1 -> Add/1
  Product10/1 -> Add4/1
  Product4/1 -> Add1/1
  SampleTime_div_Ld/1 -> Product1/1
  y_phase_voltage_per_switching_state/1 -> Subtract3/1
  Product2/1 -> Subtract/2
  Subtract5/1 -> Square1/1
  Product3/1 -> Subtract/3
  SampleTime_div_Lq/1 -> Product4/1
  Subtract/1 -> Product1/2
  Subtract3/1 -> Product10/2
  Sum of Elements/1 -> J/1  "J"
  psiPM/1 -> Add2/1
  id_ref/1 -> Subtract4/1
  Subtract6/1 -> Square2/1
  Ld/1 -> Product7/2
  iy_ref/1 -> Subtract7/1
  ix_k/1 -> Add3/2, Product9/1
  Subtract4/1 -> Square4/1
  Subtract7/1 -> Square3/1
  iq_ref/1 -> Subtract5/1
  SampleTime_div_Lx/1 -> Product8/1
  d_phase_voltage_per_switching_state/1 -> Subtract/1
  Square3/1 -> Sum of Elements/4
  Square2/1 -> Sum of Elements/3
  Square1/1 -> Sum of Elements/2
  Square4/1 -> Sum of Elements/1

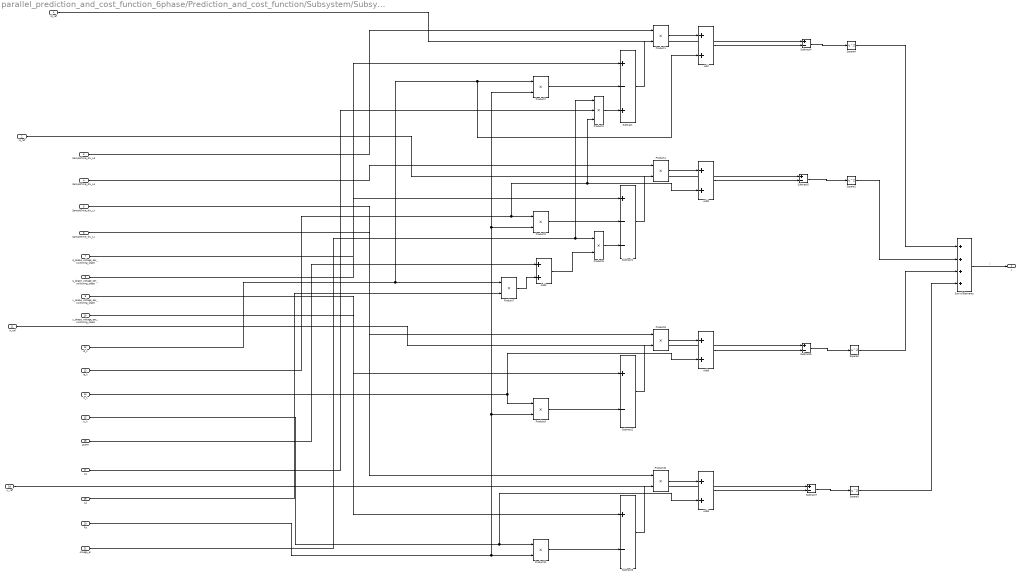
== system parallel_prediction_and_cost_function_6phase/Prediction_and_cost_function/Subsystem/Subsystem15 ==
  id_ref : Inport
  iq_ref : Inport  Port=2
  SampleTime_div_Ld : Inport  Port=3
  SampleTime_div_Lq : Inport  Port=4
  SampleTime_div_Lx : Inport  Port=5
  SampleTime_div_Ly : Inport  Port=6
  d_phase_voltage_per_switching_state : Inport  Port=7
  q_phase_voltage_per_switching_state : Inport  Port=8
  x_phase_voltage_per_switching_state : Inport  Port=9
  y_phase_voltage_per_switching_state : Inport  Port=10
  ix_ref : Inport  Port=11
  id_k : Inport  Port=12
  iq_k : Inport  Port=13
  ix_k : Inport  Port=14
  iy_k : Inport  Port=15
  psiPM : Inport  Port=16
  Lq : Inport  Port=17
  iy_ref : Inport  Port=18
  Ld : Inport  Port=19
  Rs : Inport  Port=20
  omega_el : Inport  Port=21
  Add{,1,3..4} (4 alike) : Sum  OutDataTypeStr=single
  Add2 : Sum
  Product{1..2,4..11} (10 alike) : Product  OutDataTypeStr=single
  Product3 : Product  Inputs=3  OutDataTypeStr=single
  Square{1..4} (4 alike) : Math  Operator=square  SignedPower=on  RndMeth=Zero
  Subtract : Sum  Inputs=+-+  OutDataTypeStr=single
  Subtract1 : Sum  Inputs=+--  OutDataTypeStr=single
  Subtract2 : Sum  Inputs=+-  OutDataTypeStr=single
  Subtract3 : Sum  Inputs=+-  OutDataTypeStr=single
  Subtract{4..7} (4 alike) : Sum  Inputs=+-
  Sum of Elements : Sum  Inputs=++++
  J : Outport
  wires:
  Add1/1 -> Subtract5/2
  q_phase_voltage_per_switching_state/1 -> Subtract1/1
  ix_ref/1 -> Subtract6/1
  omega_el/1 -> Product3/1, Product6/1
  Product5/1 -> Subtract1/2
  iq_k/1 -> Product3/3, Add1/2, Product5/1
  iy_k/1 -> Add4/2, Product11/1
  Add2/1 -> Product6/2
  Lq/1 -> Product3/2
  Add4/1 -> Subtract7/2
  Subtract2/1 -> Product8/2
  SampleTime_div_Ly/1 -> Product10/1
  Rs/1 -> Product9/2, Product2/2, Product5/2, Product11/2
  Product9/1 -> Subtract2/2
  Product8/1 -> Add3/1
  Product7/1 -> Add2/2
  id_k/1 -> Add/2, Product2/1, Product7/1
  x_phase_voltage_per_switching_state/1 -> Subtract2/1
  Add3/1 -> Subtract6/2
  Add/1 -> Subtract4/2
  Product11/1 -> Subtract3/2
  Product6/1 -> Subtract1/3
  Subtract1/1 -> Product4/2
  Product1/1 -> Add/1
  Product10/1 -> Add4/1
  Product4/1 -> Add1/1
  SampleTime_div_Ld/1 -> Product1/1
  y_phase_voltage_per_switching_state/1 -> Subtract3/1
  Product2/1 -> Subtract/2
  Subtract5/1 -> Square1/1
  Product3/1 -> Subtract/3
  SampleTime_div_Lq/1 -> Product4/1
  Subtract/1 -> Product1/2
  Subtract3/1 -> Product10/2
  Sum of Elements/1 -> J/1  "J"
  psiPM/1 -> Add2/1
  id_ref/1 -> Subtract4/1
  Subtract6/1 -> Square2/1
  Ld/1 -> Product7/2
  iy_ref/1 -> Subtract7/1
  ix_k/1 -> Add3/2, Product9/1
  Subtract4/1 -> Square4/1
  Subtract7/1 -> Square3/1
  iq_ref/1 -> Subtract5/1
  SampleTime_div_Lx/1 -> Product8/1
  d_phase_voltage_per_switching_state/1 -> Subtract/1
  Square3/1 -> Sum of Elements/4
  Square2/1 -> Sum of Elements/3
  Square1/1 -> Sum of Elements/2
  Square4/1 -> Sum of Elements/1

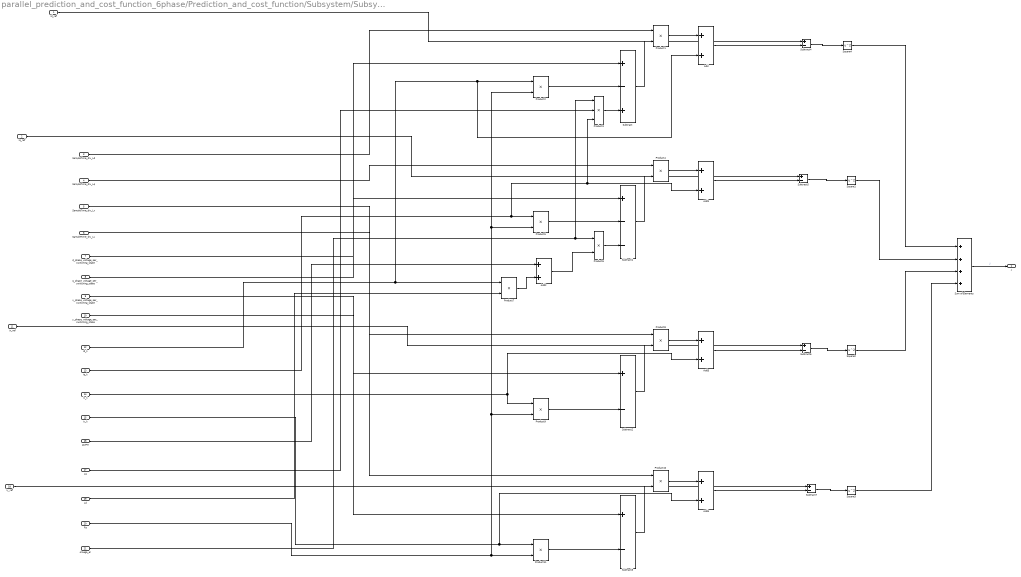
== system parallel_prediction_and_cost_function_6phase/Prediction_and_cost_function/Subsystem/Subsystem2 ==
  id_ref : Inport
  iq_ref : Inport  Port=2
  SampleTime_div_Ld : Inport  Port=3
  SampleTime_div_Lq : Inport  Port=4
  SampleTime_div_Lx : Inport  Port=5
  SampleTime_div_Ly : Inport  Port=6
  d_phase_voltage_per_switching_state : Inport  Port=7
  q_phase_voltage_per_switching_state : Inport  Port=8
  x_phase_voltage_per_switching_state : Inport  Port=9
  y_phase_voltage_per_switching_state : Inport  Port=10
  ix_ref : Inport  Port=11
  id_k : Inport  Port=12
  iq_k : Inport  Port=13
  ix_k : Inport  Port=14
  iy_k : Inport  Port=15
  psiPM : Inport  Port=16
  Lq : Inport  Port=17
  iy_ref : Inport  Port=18
  Ld : Inport  Port=19
  Rs : Inport  Port=20
  omega_el : Inport  Port=21
  Add{,1,3..4} (4 alike) : Sum  OutDataTypeStr=single
  Add2 : Sum
  Product{1..2,4..11} (10 alike) : Product  OutDataTypeStr=single
  Product3 : Product  Inputs=3  OutDataTypeStr=single
  Square{1..4} (4 alike) : Math  Operator=square  SignedPower=on  RndMeth=Zero
  Subtract : Sum  Inputs=+-+  OutDataTypeStr=single
  Subtract1 : Sum  Inputs=+--  OutDataTypeStr=single
  Subtract2 : Sum  Inputs=+-  OutDataTypeStr=single
  Subtract3 : Sum  Inputs=+-  OutDataTypeStr=single
  Subtract{4..7} (4 alike) : Sum  Inputs=+-
  Sum of Elements : Sum  Inputs=++++
  J : Outport
  wires:
  Add1/1 -> Subtract5/2
  q_phase_voltage_per_switching_state/1 -> Subtract1/1
  ix_ref/1 -> Subtract6/1
  omega_el/1 -> Product3/1, Product6/1
  Product5/1 -> Subtract1/2
  iq_k/1 -> Product3/3, Add1/2, Product5/1
  iy_k/1 -> Add4/2, Product11/1
  Add2/1 -> Product6/2
  Lq/1 -> Product3/2
  Add4/1 -> Subtract7/2
  Subtract2/1 -> Product8/2
  SampleTime_div_Ly/1 -> Product10/1
  Rs/1 -> Product9/2, Product2/2, Product5/2, Product11/2
  Product9/1 -> Subtract2/2
  Product8/1 -> Add3/1
  Product7/1 -> Add2/2
  id_k/1 -> Add/2, Product2/1, Product7/1
  x_phase_voltage_per_switching_state/1 -> Subtract2/1
  Add3/1 -> Subtract6/2
  Add/1 -> Subtract4/2
  Product11/1 -> Subtract3/2
  Product6/1 -> Subtract1/3
  Subtract1/1 -> Product4/2
  Product1/1 -> Add/1
  Product10/1 -> Add4/1
  Product4/1 -> Add1/1
  SampleTime_div_Ld/1 -> Product1/1
  y_phase_voltage_per_switching_state/1 -> Subtract3/1
  Product2/1 -> Subtract/2
  Subtract5/1 -> Square1/1
  Product3/1 -> Subtract/3
  SampleTime_div_Lq/1 -> Product4/1
  Subtract/1 -> Product1/2
  Subtract3/1 -> Product10/2
  Sum of Elements/1 -> J/1  "J"
  psiPM/1 -> Add2/1
  id_ref/1 -> Subtract4/1
  Subtract6/1 -> Square2/1
  Ld/1 -> Product7/2
  iy_ref/1 -> Subtract7/1
  ix_k/1 -> Add3/2, Product9/1
  Subtract4/1 -> Square4/1
  Subtract7/1 -> Square3/1
  iq_ref/1 -> Subtract5/1
  SampleTime_div_Lx/1 -> Product8/1
  d_phase_voltage_per_switching_state/1 -> Subtract/1
  Square3/1 -> Sum of Elements/4
  Square2/1 -> Sum of Elements/3
  Square1/1 -> Sum of Elements/2
  Square4/1 -> Sum of Elements/1

== system parallel_prediction_and_cost_function_6phase/Prediction_and_cost_function/Subsystem/Subsystem3 ==
  id_ref : Inport
  iq_ref : Inport  Port=2
  SampleTime_div_Ld : Inport  Port=3
  SampleTime_div_Lq : Inport  Port=4
  SampleTime_div_Lx : Inport  Port=5
  SampleTime_div_Ly : Inport  Port=6
  d_phase_voltage_per_switching_state : Inport  Port=7
  q_phase_voltage_per_switching_state : Inport  Port=8
  x_phase_voltage_per_switching_state : Inport  Port=9
  y_phase_voltage_per_switching_state : Inport  Port=10
  ix_ref : Inport  Port=11
  id_k : Inport  Port=12
  iq_k : Inport  Port=13
  ix_k : Inport  Port=14
  iy_k : Inport  Port=15
  psiPM : Inport  Port=16
  Lq : Inport  Port=17
  iy_ref : Inport  Port=18
  Ld : Inport  Port=19
  Rs : Inport  Port=20
  omega_el : Inport  Port=21
  Add{,1,3..4} (4 alike) : Sum  OutDataTypeStr=single
  Add2 : Sum
  Product{1..2,4..11} (10 alike) : Product  OutDataTypeStr=single
  Product3 : Product  Inputs=3  OutDataTypeStr=single
  Square{1..4} (4 alike) : Math  Operator=square  SignedPower=on  RndMeth=Zero
  Subtract : Sum  Inputs=+-+  OutDataTypeStr=single
  Subtract1 : Sum  Inputs=+--  OutDataTypeStr=single
  Subtract2 : Sum  Inputs=+-  OutDataTypeStr=single
  Subtract3 : Sum  Inputs=+-  OutDataTypeStr=single
  Subtract{4..7} (4 alike) : Sum  Inputs=+-
  Sum of Elements : Sum  Inputs=++++
  J : Outport
  wires:
  Add1/1 -> Subtract5/2
  q_phase_voltage_per_switching_state/1 -> Subtract1/1
  ix_ref/1 -> Subtract6/1
  omega_el/1 -> Product3/1, Product6/1
  Product5/1 -> Subtract1/2
  iq_k/1 -> Product3/3, Add1/2, Product5/1
  iy_k/1 -> Add4/2, Product11/1
  Add2/1 -> Product6/2
  Lq/1 -> Product3/2
  Add4/1 -> Subtract7/2
  Subtract2/1 -> Product8/2
  SampleTime_div_Ly/1 -> Product10/1
  Rs/1 -> Product9/2, Product2/2, Product5/2, Product11/2
  Product9/1 -> Subtract2/2
  Product8/1 -> Add3/1
  Product7/1 -> Add2/2
  id_k/1 -> Add/2, Product2/1, Product7/1
  x_phase_voltage_per_switching_state/1 -> Subtract2/1
  Add3/1 -> Subtract6/2
  Add/1 -> Subtract4/2
  Product11/1 -> Subtract3/2
  Product6/1 -> Subtract1/3
  Subtract1/1 -> Product4/2
  Product1/1 -> Add/1
  Product10/1 -> Add4/1
  Product4/1 -> Add1/1
  SampleTime_div_Ld/1 -> Product1/1
  y_phase_voltage_per_switching_state/1 -> Subtract3/1
  Product2/1 -> Subtract/2
  Subtract5/1 -> Square1/1
  Product3/1 -> Subtract/3
  SampleTime_div_Lq/1 -> Product4/1
  Subtract/1 -> Product1/2
  Subtract3/1 -> Product10/2
  Sum of Elements/1 -> J/1  "J"
  psiPM/1 -> Add2/1
  id_ref/1 -> Subtract4/1
  Subtract6/1 -> Square2/1
  Ld/1 -> Product7/2
  iy_ref/1 -> Subtract7/1
  ix_k/1 -> Add3/2, Product9/1
  Subtract4/1 -> Square4/1
  Subtract7/1 -> Square3/1
  iq_ref/1 -> Subtract5/1
  SampleTime_div_Lx/1 -> Product8/1
  d_phase_voltage_per_switching_state/1 -> Subtract/1
  Square3/1 -> Sum of Elements/4
  Square2/1 -> Sum of Elements/3
  Square1/1 -> Sum of Elements/2
  Square4/1 -> Sum of Elements/1
